simulink model "PubIfDecisionTOS_MDL"  (R2020b)
settings: configuration reference "DspaceConfig" (kept outside this file)
PostLoadFcn:
  | if any(exist('dsrtsu_mdlpostloadfcn', 'file') ~= 0), dsrtsu_mdlpostloadfcn('Execute', bdroot); end
InitFcn:
  | , if any(exist('dsmpb_private', 'file') ~= 0), dsmpb_private('dsmpb_mdlclblib', 'Init', bdroot); end,
undefined symbols (not defined in the file or in its folder): C_TOS_ACCEgoRAxletoFbumplength_m, C_TOS_ACCTargetFront_Flag, C_TOS_AEBJAPedObjDxThre_Val, C_TOS_AEBJAPedObjDyThre_Val, C_TOS_AEBJATargetSize_Val, C_TOS_AEBJAVehObjDxThre_Val, C_TOS_AEBJAVehObjDyThre_Val, C_TOS_AEBJuncPedTargetSize_Val, C_TOS_AEBLatObjDxThre_Val, C_TOS_AEBLatPedDyThre_Val, C_TOS_AEBLatTargetSize_Val, C_TOS_AEBLongTargetInEgoFront_Flag, C_TOS_axAbsGround_Parameter, C_TOS_CameraConfirmedFlag, C_TOS_CNsubjWidth, C_TOS_CurrentLaneCoreMinWidth_Val, C_TOS_CutInProb_Val_Zero, C_TOS_CutOutProb_Val_Zero, C_TOS_D2R_Val, C_TOS_DefaultValueObjectToCenterLine_dy, C_TOS_EgoCarWidth_Val, C_TOS_EgoDxRefPoint_m, C_TOS_EgoRAxletoFbumplength_m, C_TOS_HalfWidthVehicle_Con, C_TOS_HWA_CurrentLaneFlag, C_TOS_HWA_LeftLaneFlag, C_TOS_HWA_MovingDir_Vaild, C_TOS_HWA_MovState_Vaild, C_TOS_HWA_RightLaneFlag, C_TOS_LaneLineCourseErrorFront, C_TOS_LaneLineCourseErrorRear, C_TOS_MotorbikeDefaultWidth_m, C_TOS_NumberOfEffectiveTargets, C_TOS_Obj_Age_Val, C_TOS_Objdx_Constraint_Val, C_TOS_ObjectDefaultWidth_m, C_TOS_ObjInCurrentLane_Val, C_TOS_ObjInCurrentLaneValid, C_TOS_ObjInLeftLaneValid, C_TOS_ObjInRightLaneValid, C_TOS_ObjNotInCurrentLane_Val, C_TOS_ObjNotREElementType, C_TOS_ObjPredictDis_dy_ConstantVal_Zeros, C_TOS_ObjToCenterLine_ConstantVal_Zeros, C_TOS_OFMObjIDInvilad_Val, C_TOS_PIL_LatDisCons_Val_zero, C_TOS_PIL_ObjectCutInFlag_b, C_TOS_PIL_ObjectCutOutFlag_b, C_TOS_PIL_ObjLaneProb_al_Val, C_TOS_PP_ObjFusType_FC_Confirm_b, C_TOS_PP_ObjFusType_FC_FR_Confirm_b, C_TOS_PP_ObjFusType_FR_Confirm_b, C_TOS_RE_80BoolDefault_Val, C_TOS_RE_80Single181Default_Val, C_TOS_RE_80Single255Default_Val, C_TOS_RE_80Uint8Default_Val, C_TOS_RE_D2R, C_TOS_RE_D_180_Val, C_TOS_RE_InvalidObjectID_Val, C_TOS_RE_InvalidTargetChainDir_Val ... (+142)
libraries: simulink x1650, TOS_LIB x361, canfdmsglib x14
(part 35 of 69)

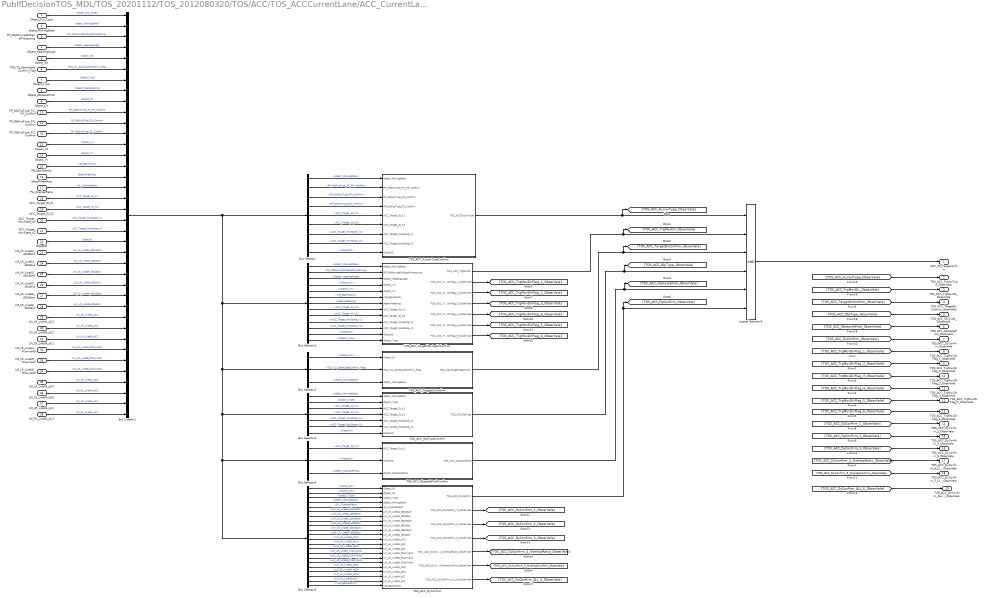
== system PubIfDecisionTOS_MDL/TOS_20201112/TOS_2012080320/TOS/ACC/TOS_ACCCurrentLane/ACC_CurrentLane_Target/TOS_ACC_P0/ACC_P0_Targe/ACC_P0_Targe ==
  Object_Fus_Type : Inport
  object_MovingState : Inport  Port=2
  PP_ObjMovingDirSignalProcessing : Inport  Port=3
  Object_HeadingAngle : Inport  Port=4
  Object_DX : Inport  Port=5
  TOS_TLJ_SameLaneConfirm_Flag : Inport  Port=6
  Object_Type : Inport  Port=7
  Object_ObstacleProb : Inport  Port=8
  Object_DY : Inport  Port=9
  PP_ObjFusType_FC_FR_Confirm : Inport  Port=10
  PP_ObjFusType_FR_Confirm : Inport  Port=11
  PP_ObjFusType_FC_Confirm : Inport  Port=12
  Object_VX : Inport  Port=13
  Object_VY : Inport  Port=14
  VIE_EgoVelocity : Inport  Port=15
  SteerWheelAng : Inport  Port=16
  PIL_OverlapRatio : Inport  Port=17
  ACC_Target_ID_K1 : Inport  Port=18
  ACC_Target_ID_K2 : Inport  Port=19
  ACC_Target_MovState_K1 : Inport  Port=20
  ACC_Target_MovState_K2 : Inport  Port=21
  ObjectID : Inport  Port=22
  LM_LR_Line04_dDisStart : Inport  Port=23
  LM_LR_Line04_dDisEnd : Inport  Port=24
  LM_LR_Line05_dDisStart : Inport  Port=25
  LM_LR_Line05_dDisEnd : Inport  Port=26
  LM_LR_Line06_dDisStart : Inport  Port=27
  LM_LR_Line06_dDisEnd : Inport  Port=28
  LM_LR_Line04_pC2 : Inport  Port=29
  LM_LR_Line05_pC2 : Inport  Port=30
  LM_LR_Line06_pC2 : Inport  Port=31
  LM_LR_Line04_fCamValid : Inport  Port=32
  LM_LR_Line05_fCamValid : Inport  Port=33
  LM_LR_Line06_fCamValid : Inport  Port=34
  LM_LR_Line04_pC0 : Inport  Port=35
  LM_RL_Line04_pC0 : Inport  Port=36
  LM_LR_Line04_pC1 : Inport  Port=37
  LM_RL_Line04_pC1 : Inport  Port=38
  Bus Creator1 : BusCreator  Inputs=38
  Bus Selector : BusSelector  OutputSignals=object_MovingState,PP_ObjFusType_FC_FR_Confirm,PP_ObjFusType_FR_Confirm,PP_ObjFusType_FC_Confirm,ACC_Target_ID_K1,ACC_Target_ID_K2,ACC_Target_MovState_K1,ACC_Target_MovState_K2,ObjectID
  Bus Selector1 : BusSelector  OutputSignals=object_MovingState,PP_ObjMovingDirSignalProcessing,Object_HeadingAngle,Object_VX,Object_VY,VIE_EgoVelocity,SteerWheelAng,ACC_Target_ID_K1,ACC_Target_ID_K2,ACC_Target_MovState_K1,ACC_Target_MovState_K2,ObjectID,Object_Type
  Bus Selector2 : BusSelector  OutputSignals=Object_DX,TOS_TLJ_SameLaneConfirm_Flag,object_MovingState
  Bus Selector3 : BusSelector  OutputSignals=object_MovingState,Object_Type,ACC_Target_ID_K1,ACC_Target_ID_K2,ACC_Target_MovState_K1,ACC_Target_MovState_K2,ObjectID
  Bus Selector4 : BusSelector  OutputSignals=ACC_Target_ID_K1,ObjectID,Object_ObstacleProb
  Bus Selector5 : BusSelector  OutputSignals=Object_DY,Object_DX,Object_Type,object_MovingState,PIL_OverlapRatio,LM_LR_Line04_dDisStart,LM_LR_Line04_dDisEnd,LM_LR_Line05_dDisStart,LM_LR_Line05_dDisEnd,LM_LR_Line06_dDisStart,LM_LR_Line06_dDisEnd,LM_LR_Line04_pC2,LM_LR_Line05_pC2,LM_LR_Line06_pC2,LM_LR_Line04_fCamValid,LM_LR_Line05_fCamValid,LM_LR_Line06_fCamValid,LM_LR_Line04_pC0,LM_RL_Line04_pC0,LM_LR_Line04_pC1,LM_RL_Line04_pC1,VIE_EgoVelocity
  Logical Operator4 : Logic  Inputs=6  AllPortsSameDT=off  OutDataTypeStr=boolean
  TOS_ACC_DyConfirm : Subsystem
  TOS_ACC_FusionTypeConfirm : Subsystem
  TOS_ACC_ObjTypeConfirm : Subsystem
  TOS_ACC_ObstacleProbConfirm : Subsystem
  TOS_ACC_TargetDxConfirm : Subsystem
  TOS_ACC_TargetMovingDirConfirm : Subsystem
  ACC_P0_TargeConfirm : Outport
  TOS_ACC_FusionType_ObserVale : Outport  Port=2
  TOS_ACC_TrgMovDir_ObserVale : Outport  Port=3
  TOS_ACC_TargetDxConfirm_ObserVale : Outport  Port=4
  TOS_ACC_ObjType_ObserVale : Outport  Port=5
  TOS_ACC_ObstacleProb_ObserVale : Outport  Port=6
  TOS_ACC_DyConfirm_ObserVale : Outport  Port=7
  TOS_ACC_TrgMovDirFlag_1_ObserVale : Outport  Port=8
  TOS_ACC_TrgMovDirFlag_2_ObserVale : Outport  Port=9
  TOS_ACC_TrgMovDirFlag_3_ObserVale : Outport  Port=10
  TOS_ACC_TrgMovDirFlag_4_ObserVale : Outport  Port=11
  TOS_ACC_TrgMovDirFlag_5_ObserVale : Outport  Port=12
  TOS_ACC_TrgMovDirFlag_6_ObserVale : Outport  Port=13
  TOS_ACC_DyConfirm_1_ObserVale : Outport  Port=14
  TOS_ACC_DyConfirm_2_ObserVale : Outport  Port=15
  TOS_ACC_DyConfirm_3_ObserVale : Outport  Port=16
  TOS_ACC_DyConfirm_4_OverlapRatio_ObserVale : Outport  Port=17
  TOS_ACC_DyConfirm_5_OverlapConfirm_ObserVale : Outport  Port=18
  TOS_ACC_DyConfirm_ALL_6_ObserVale : Outport  Port=19
  wires:
  Bus Selector2/2 -> TOS_ACC_TargetDxConfirm/2(TOS_TLJ_SameLaneConfirm_Flag)  "<TOS_TLJ_SameLaneConfirm_Flag>"
  TOS_ACC_TargetDxConfirm/1(TOS_ACCTargetInEgoFront) -> [TOS_ACC_TargetDxConfirm_ObserVale], Logical Operator4/3
  TOS_ACC_TargetMovingDirConfirm/1(TOS_ACC_TrgMovDir) -> [TOS_ACC_TrgMovDir_ObserVale], Logical Operator4/2
  Bus Selector2/1 -> TOS_ACC_TargetDxConfirm/1(Object_Dx)  "<Object_DX>"
  TOS_ACC_FusionTypeConfirm/1(TOS_ACCFusionType) -> [TOS_ACC_FusionType_ObserVale], Logical Operator4/1
  TOS_ACC_ObjTypeConfirm/1(TOS_ACCObjType) -> Logical Operator4/4, [TOS_ACC_ObjType_ObserVale]
  Logical Operator4/1 -> ACC_P0_TargeConfirm/1
  [TOS_ACC_FusionType_ObserVale] -> TOS_ACC_FusionType_ObserVale/1
  [TOS_ACC_TrgMovDir_ObserVale] -> TOS_ACC_TrgMovDir_ObserVale/1
  [TOS_ACC_TargetDxConfirm_ObserVale] -> TOS_ACC_TargetDxConfirm_ObserVale/1
  [TOS_ACC_ObjType_ObserVale] -> TOS_ACC_ObjType_ObserVale/1
  [TOS_ACC_ObstacleProb_ObserVale] -> TOS_ACC_ObstacleProb_ObserVale/1
  Bus Selector/1 -> TOS_ACC_FusionTypeConfirm/1(object_MovingState)  "<object_MovingState>"
  Bus Selector1/1 -> TOS_ACC_TargetMovingDirConfirm/1(object_MovingState)  "<object_MovingState>"
  Bus Selector4/3 -> TOS_ACC_ObstacleProbConfirm/3(Object_ObstacleProb)  "<Object_ObstacleProb>"
  TOS_ACC_ObstacleProbConfirm/1(TOS_ACC_ObstacleProb) -> Logical Operator4/5, [TOS_ACC_ObstacleProb_ObserVale]
  TOS_ACC_DyConfirm/1(TOS_ACC_DyConfirm) -> [TOS_ACC_DyConfirm_ObserVale], Logical Operator4/6
  [TOS_ACC_DyConfirm_ObserVale] -> TOS_ACC_DyConfirm_ObserVale/1
  Bus Selector/2 -> TOS_ACC_FusionTypeConfirm/2(PP_ObjFusType_FC_FR_Confirm)  "<PP_ObjFusType_FC_FR_Confirm>"
  Bus Selector/3 -> TOS_ACC_FusionTypeConfirm/3(PP_ObjFusType_FR_Confirm)  "<PP_ObjFusType_FR_Confirm>"
  Bus Selector/4 -> TOS_ACC_FusionTypeConfirm/4(PP_ObjFusType_FC_Confirm)  "<PP_ObjFusType_FC_Confirm>"
  [TOS_ACC_DyConfirm_4_OverlapRatio_ObserVale] -> TOS_ACC_DyConfirm_4_OverlapRatio_ObserVale/1
  Bus Selector/5 -> TOS_ACC_FusionTypeConfirm/5(ACC_Target_ID_K1)  "<ACC_Target_ID_K1>"
  Bus Selector/6 -> TOS_ACC_FusionTypeConfirm/6(ACC_Target_ID_K2)  "<ACC_Target_ID_K2>"
  Bus Selector/9 -> TOS_ACC_FusionTypeConfirm/9(ObjectID)  "<ObjectID>"
  Object_DY/1 -> Bus Creator1/9  "Object_DY"
  PP_ObjFusType_FC_Confirm/1 -> Bus Creator1/12  "PP_ObjFusType_FC_Confirm"
  PP_ObjFusType_FR_Confirm/1 -> Bus Creator1/11  "PP_ObjFusType_FR_Confirm"
  SteerWheelAng/1 -> Bus Creator1/16  "SteerWheelAng"
  PIL_OverlapRatio/1 -> Bus Creator1/17  "PIL_OverlapRatio"
  ACC_Target_MovState_K1/1 -> Bus Creator1/20  "ACC_Target_MovState_K1"
  ACC_Target_ID_K2/1 -> Bus Creator1/19  "ACC_Target_ID_K2"
  Object_DX/1 -> Bus Creator1/5  "Object_DX"
  Object_ObstacleProb/1 -> Bus Creator1/8  "Object_ObstacleProb"
  ObjectID/1 -> Bus Creator1/22  "ObjectID"
  PP_ObjMovingDirSignalProcessing/1 -> Bus Creator1/3  "PP_ObjMovingDirSignalProcessing"
  VIE_EgoVelocity/1 -> Bus Creator1/15  "VIE_EgoVelocity"
  ACC_Target_ID_K1/1 -> Bus Creator1/18  "ACC_Target_ID_K1"
  Object_HeadingAngle/1 -> Bus Creator1/4  "Object_HeadingAngle"
  PP_ObjFusType_FC_FR_Confirm/1 -> Bus Creator1/10  "PP_ObjFusType_FC_FR_Confirm"
  object_MovingState/1 -> Bus Creator1/2  "object_MovingState"
  ACC_Target_MovState_K2/1 -> Bus Creator1/21  "ACC_Target_MovState_K2"
  Object_VY/1 -> Bus Creator1/14  "Object_VY"
  Object_Fus_Type/1 -> Bus Creator1/1  "Object_Fus_Type1"
  Object_Type/1 -> Bus Creator1/7  "Object_Type"
  Object_VX/1 -> Bus Creator1/13  "Object_VX"
  TOS_TLJ_SameLaneConfirm_Flag/1 -> Bus Creator1/6  "TOS_TLJ_SameLaneConfirm_Flag"
  Bus Creator1/1 -> Bus Selector5/1, Bus Selector4/1, Bus Selector3/1, Bus Selector2/1, Bus Selector1/1, Bus Selector/1
  Bus Selector/7 -> TOS_ACC_FusionTypeConfirm/7(ACC_Target_MovState_K1)  "<ACC_Target_MovState_K1>"
  Bus Selector/8 -> TOS_ACC_FusionTypeConfirm/8(ACC_Target_MovState_K2)  "<ACC_Target_MovState_K2>"
  Bus Selector1/2 -> TOS_ACC_TargetMovingDirConfirm/2(PP_ObjMovingDirSignalProcessing)  "<PP_ObjMovingDirSignalProcessing>"
  Bus Selector1/3 -> TOS_ACC_TargetMovingDirConfirm/3(Object_HeadingAngle)  "<Object_HeadingAngle>"
  Bus Selector1/4 -> TOS_ACC_TargetMovingDirConfirm/4(Object_VX)  "<Object_VX>"
  Bus Selector1/5 -> TOS_ACC_TargetMovingDirConfirm/5(Object_VY)  "<Object_VY>"
  Bus Selector1/6 -> TOS_ACC_TargetMovingDirConfirm/6(VIE_EgoVelocity)  "<VIE_EgoVelocity>"
  Bus Selector1/7 -> TOS_ACC_TargetMovingDirConfirm/7(SteerWheelAng)  "<SteerWheelAng>"
  Bus Selector3/1 -> TOS_ACC_ObjTypeConfirm/1(object_MovingState)  "<object_MovingState>"
  Bus Selector3/2 -> TOS_ACC_ObjTypeConfirm/2(Object_Type)  "<Object_Type>"
  Bus Selector5/1 -> TOS_ACC_DyConfirm/1(Object_DY)  "<Object_DY>"
  Bus Selector5/2 -> TOS_ACC_DyConfirm/2(Object_DX)  "<Object_DX>"
  Bus Selector5/3 -> TOS_ACC_DyConfirm/3(Object_Type)  "<Object_Type>"
  Bus Selector4/1 -> TOS_ACC_ObstacleProbConfirm/1(ACC_Target_ID_K1)  "<ACC_Target_ID_K1>"
  Bus Selector4/2 -> TOS_ACC_ObstacleProbConfirm/2(ObjectID)  "<ObjectID>"
  Bus Selector3/3 -> TOS_ACC_ObjTypeConfirm/3(ACC_Target_ID_K1)  "<ACC_Target_ID_K1>"
  Bus Selector3/4 -> TOS_ACC_ObjTypeConfirm/4(ACC_Target_ID_K2)  "<ACC_Target_ID_K2>"
  Bus Selector3/5 -> TOS_ACC_ObjTypeConfirm/5(ACC_Target_MovState_K1)  "<ACC_Target_MovState_K1>"
  Bus Selector3/6 -> TOS_ACC_ObjTypeConfirm/6(ACC_Target_MovState_K2)  "<ACC_Target_MovState_K2>"
  Bus Selector3/7 -> TOS_ACC_ObjTypeConfirm/7(ObjectID)  "<ObjectID>"
  Bus Selector1/8 -> TOS_ACC_TargetMovingDirConfirm/8(ACC_Target_ID_K1)  "<ACC_Target_ID_K1>"
  Bus Selector1/9 -> TOS_ACC_TargetMovingDirConfirm/9(ACC_Target_ID_K2)  "<ACC_Target_ID_K2>"
  Bus Selector1/10 -> TOS_ACC_TargetMovingDirConfirm/10(ACC_Target_MovState_K1)  "<ACC_Target_MovState_K1>"
  Bus Selector1/11 -> TOS_ACC_TargetMovingDirConfirm/11(ACC_Target_MovState_K2)  "<ACC_Target_MovState_K2>"
  Bus Selector1/12 -> TOS_ACC_TargetMovingDirConfirm/12(ObjectID)  "<ObjectID>"
  [TOS_ACC_TrgMovDirFlag_1_ObserVale] -> TOS_ACC_TrgMovDirFlag_1_ObserVale/1
  [TOS_ACC_TrgMovDirFlag_3_ObserVale] -> TOS_ACC_TrgMovDirFlag_3_ObserVale/1
  [TOS_ACC_TrgMovDirFlag_2_ObserVale] -> TOS_ACC_TrgMovDirFlag_2_ObserVale/1
  [TOS_ACC_TrgMovDirFlag_5_ObserVale] -> TOS_ACC_TrgMovDirFlag_5_ObserVale/1
  [TOS_ACC_TrgMovDirFlag_4_ObserVale] -> TOS_ACC_TrgMovDirFlag_4_ObserVale/1
  TOS_ACC_TargetMovingDirConfirm/2(TOS_ACC_TrgMovDirFlag_1_ObserVale) -> [TOS_ACC_TrgMovDirFlag_1_ObserVale]
  TOS_ACC_TargetMovingDirConfirm/3(TOS_ACC_TrgMovDirFlag_2_ObserVale) -> [TOS_ACC_TrgMovDirFlag_2_ObserVale]
  TOS_ACC_TargetMovingDirConfirm/4(TOS_ACC_TrgMovDirFlag_3_ObserVale) -> [TOS_ACC_TrgMovDirFlag_3_ObserVale]
  TOS_ACC_TargetMovingDirConfirm/5(TOS_ACC_TrgMovDirFlag_4_ObserVale) -> [TOS_ACC_TrgMovDirFlag_4_ObserVale]
  TOS_ACC_TargetMovingDirConfirm/6(TOS_ACC_TrgMovDirFlag_5_ObserVale) -> [TOS_ACC_TrgMovDirFlag_5_ObserVale]
  Bus Selector2/3 -> TOS_ACC_TargetDxConfirm/3(object_MovingState)  "<object_MovingState>"
  Bus Selector5/4 -> TOS_ACC_DyConfirm/4(object_MovingState)  "<object_MovingState>"
  [TOS_ACC_DyConfirm_2_ObserVale] -> TOS_ACC_DyConfirm_2_ObserVale/1
  [TOS_ACC_DyConfirm_3_ObserVale] -> TOS_ACC_DyConfirm_3_ObserVale/1
  [TOS_ACC_DyConfirm_1_ObserVale] -> TOS_ACC_DyConfirm_1_ObserVale/1
  TOS_ACC_DyConfirm/2(TOS_ACC_DyConfirm_1_ObserVale) -> [TOS_ACC_DyConfirm_1_ObserVale]
  TOS_ACC_DyConfirm/3(TOS_ACC_DyConfirm_2_ObserVale) -> [TOS_ACC_DyConfirm_2_ObserVale]
  TOS_ACC_DyConfirm/4(TOS_ACC_DyConfirm_3_ObserVale) -> [TOS_ACC_DyConfirm_3_ObserVale]
  TOS_ACC_TargetMovingDirConfirm/7(TOS_ACC_TrgMovDirFlag_6_ObserVale) -> [TOS_ACC_TrgMovDirFlag_6_ObserVale]
  [TOS_ACC_TrgMovDirFlag_6_ObserVale] -> TOS_ACC_TrgMovDirFlag_6_ObserVale/1
  Bus Selector5/5 -> TOS_ACC_DyConfirm/5(PIL_OverlapRatio)  "<PIL_OverlapRatio>"
  TOS_ACC_DyConfirm/5(TOS_ACC_DyConfirm_4_OverlapRatio_ObserVale) -> [TOS_ACC_DyConfirm_4_OverlapRatio_ObserVale]
  Bus Selector1/13 -> TOS_ACC_TargetMovingDirConfirm/13(Object_Type)  "<Object_Type>"
  LM_LR_Line04_dDisStart/1 -> Bus Creator1/23  "LM_LR_Line04_dDisStart"
  LM_LR_Line04_dDisEnd/1 -> Bus Creator1/24  "LM_LR_Line04_dDisEnd"
  LM_LR_Line05_dDisStart/1 -> Bus Creator1/25  "LM_LR_Line05_dDisStart"
  LM_LR_Line05_dDisEnd/1 -> Bus Creator1/26  "LM_LR_Line05_dDisEnd"
  LM_LR_Line06_dDisStart/1 -> Bus Creator1/27  "LM_LR_Line06_dDisStart"
  LM_LR_Line06_dDisEnd/1 -> Bus Creator1/28  "LM_LR_Line06_dDisEnd"
  LM_LR_Line04_pC2/1 -> Bus Creator1/29  "LM_LR_Line04_pC2"
  LM_LR_Line05_pC2/1 -> Bus Creator1/30  "LM_LR_Line05_pC2"
  LM_LR_Line06_pC2/1 -> Bus Creator1/31  "LM_LR_Line06_pC2"
  Bus Selector5/6 -> TOS_ACC_DyConfirm/6(LM_LR_Line04_dDisStart)  "<LM_LR_Line04_dDisStart>"
  Bus Selector5/7 -> TOS_ACC_DyConfirm/7(LM_LR_Line04_dDisEnd)  "<LM_LR_Line04_dDisEnd>"
  Bus Selector5/8 -> TOS_ACC_DyConfirm/8(LM_LR_Line05_dDisStart)  "<LM_LR_Line05_dDisStart>"
  Bus Selector5/9 -> TOS_ACC_DyConfirm/9(LM_LR_Line05_dDisEnd)  "<LM_LR_Line05_dDisEnd>"
  Bus Selector5/10 -> TOS_ACC_DyConfirm/10(LM_LR_Line06_dDisStart)  "<LM_LR_Line06_dDisStart>"
  Bus Selector5/11 -> TOS_ACC_DyConfirm/11(LM_LR_Line06_dDisEnd)  "<LM_LR_Line06_dDisEnd>"
  Bus Selector5/12 -> TOS_ACC_DyConfirm/12(LM_LR_Line04_pC2)  "<LM_LR_Line04_pC2>"
  Bus Selector5/13 -> TOS_ACC_DyConfirm/13(LM_LR_Line05_pC2)  "<LM_LR_Line05_pC2>"
  Bus Selector5/14 -> TOS_ACC_DyConfirm/14(LM_LR_Line06_pC2)  "<LM_LR_Line06_pC2>"
  LM_LR_Line04_fCamValid/1 -> Bus Creator1/32  "LM_LR_Line04_fCamValid"
  LM_LR_Line05_fCamValid/1 -> Bus Creator1/33  "LM_LR_Line05_fCamValid"
  LM_LR_Line06_fCamValid/1 -> Bus Creator1/34  "LM_LR_Line06_fCamValid"
  Bus Selector5/15 -> TOS_ACC_DyConfirm/15(LM_LR_Line04_fCamValid)  "<LM_LR_Line04_fCamValid>"
  Bus Selector5/16 -> TOS_ACC_DyConfirm/16(LM_LR_Line05_fCamValid)  "<LM_LR_Line05_fCamValid>"
  Bus Selector5/17 -> TOS_ACC_DyConfirm/17(LM_LR_Line06_fCamValid)  "<LM_LR_Line06_fCamValid>"
  [TOS_ACC_DyConfirm_5_OverlapConfirm_ObserVale] -> TOS_ACC_DyConfirm_5_OverlapConfirm_ObserVale/1
  TOS_ACC_DyConfirm/6(TOS_ACC_DyConfirm_5_OverlapConfirm_ObserVale) -> [TOS_ACC_DyConfirm_5_OverlapConfirm_ObserVale]
  TOS_ACC_DyConfirm/7(TOS_ACC_DyConfirm_ALL_6_ObserVale) -> [TOS_ACC_DyConfirm_ALL_6_ObserVale]
  [TOS_ACC_DyConfirm_ALL_6_ObserVale] -> TOS_ACC_DyConfirm_ALL_6_ObserVale/1
  LM_LR_Line04_pC0/1 -> Bus Creator1/35  "LM_LR_Line04_pC0"
  LM_RL_Line04_pC0/1 -> Bus Creator1/36  "LM_RL_Line04_pC0"
  Bus Selector5/18 -> TOS_ACC_DyConfirm/18(LM_LR_Line04_pC0)  "<LM_LR_Line04_pC0>"
  Bus Selector5/19 -> TOS_ACC_DyConfirm/19(LM_RL_Line04_pC0)  "<LM_RL_Line04_pC0>"
  LM_LR_Line04_pC1/1 -> Bus Creator1/37  "LM_LR_Line04_pC1"
  LM_RL_Line04_pC1/1 -> Bus Creator1/38  "LM_RL_Line04_pC1"
  Bus Selector5/20 -> TOS_ACC_DyConfirm/20(LM_LR_Line04_pC1)  "<LM_LR_Line04_pC1>"
  Bus Selector5/21 -> TOS_ACC_DyConfirm/21(LM_RL_Line04_pC1)  "<LM_RL_Line04_pC1>"
  Bus Selector5/22 -> TOS_ACC_DyConfirm/22(VIE_EgoVelocity)  "<VIE_EgoVelocity>"

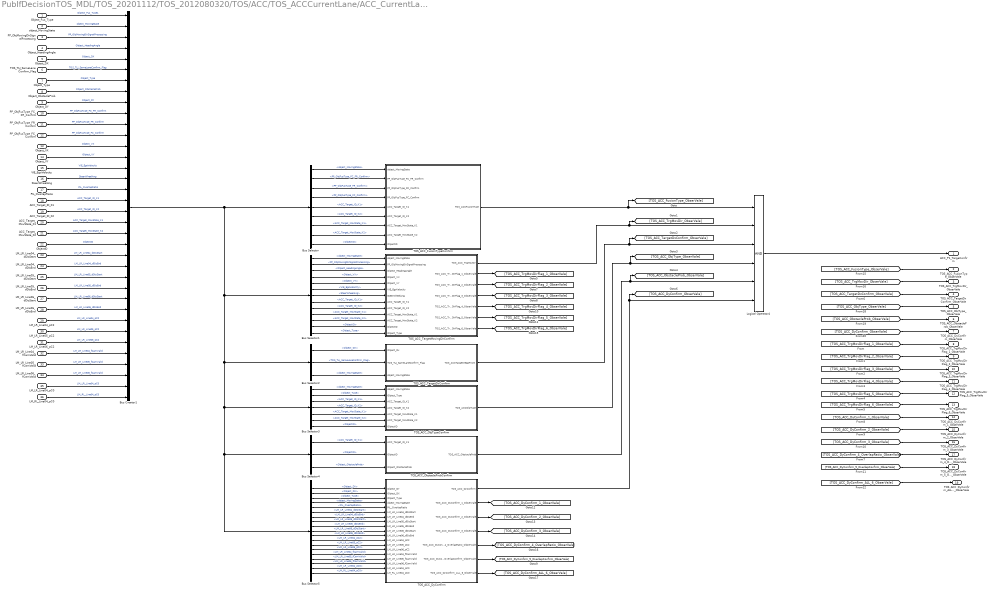
== system PubIfDecisionTOS_MDL/TOS_20201112/TOS_2012080320/TOS/ACC/TOS_ACCCurrentLane/ACC_CurrentLane_Target/TOS_ACC_P1/ACC_P1_Targe/ACC_P1_Targe ==
  Object_Fus_Type : Inport
  object_MovingState : Inport  Port=2
  PP_ObjMovingDirSignalProcessing : Inport  Port=3
  Object_HeadingAngle : Inport  Port=4
  Object_DX : Inport  Port=5
  TOS_TLJ_SameLaneConfirm_Flag : Inport  Port=6
  Object_Type : Inport  Port=7
  Object_ObstacleProb : Inport  Port=8
  Object_DY : Inport  Port=9
  PP_ObjFusType_FC_FR_Confirm : Inport  Port=10
  PP_ObjFusType_FR_Confirm : Inport  Port=11
  PP_ObjFusType_FC_Confirm : Inport  Port=12
  Object_VX : Inport  Port=13
  Object_VY : Inport  Port=14
  VIE_EgoVelocity : Inport  Port=15
  SteerWheelAng : Inport  Port=16
  PIL_OverlapRatio : Inport  Port=17
  ACC_Target_ID_K1 : Inport  Port=18
  ACC_Target_ID_K2 : Inport  Port=19
  ACC_Target_MovState_K1 : Inport  Port=20
  ACC_Target_MovState_K2 : Inport  Port=21
  ObjectID : Inport  Port=22
  LM_LR_Line04_dDisStart : Inport  Port=23
  LM_LR_Line04_dDisEnd : Inport  Port=24
  LM_LR_Line05_dDisStart : Inport  Port=25
  LM_LR_Line05_dDisEnd : Inport  Port=26
  LM_LR_Line06_dDisStart : Inport  Port=27
  LM_LR_Line06_dDisEnd : Inport  Port=28
  LM_LR_Line04_pC2 : Inport  Port=29
  LM_LR_Line05_pC2 : Inport  Port=30
  LM_LR_Line06_pC2 : Inport  Port=31
  LM_LR_Line04_fCamValid : Inport  Port=32
  LM_LR_Line05_fCamValid : Inport  Port=33
  LM_LR_Line06_fCamValid : Inport  Port=34
  LM_LR_Line04_pC0 : Inport  Port=35
  LM_RL_Line04_pC0 : Inport  Port=36
  Bus Creator1 : BusCreator  Inputs=36
  Bus Selector : BusSelector  OutputSignals=object_MovingState,PP_ObjFusType_FC_FR_Confirm,PP_ObjFusType_FR_Confirm,PP_ObjFusType_FC_Confirm,ACC_Target_ID_K1,ACC_Target_ID_K2,ACC_Target_MovState_K1,ACC_Target_MovState_K2,ObjectID
  Bus Selector1 : BusSelector  OutputSignals=object_MovingState,PP_ObjMovingDirSignalProcessing,Object_HeadingAngle,Object_VX,Object_VY,VIE_EgoVelocity,SteerWheelAng,ACC_Target_ID_K1,ACC_Target_ID_K2,ACC_Target_MovState_K1,ACC_Target_MovState_K2,ObjectID,Object_Type
  Bus Selector2 : BusSelector  OutputSignals=Object_DX,TOS_TLJ_SameLaneConfirm_Flag,object_MovingState
  Bus Selector3 : BusSelector  OutputSignals=object_MovingState,Object_Type,ACC_Target_ID_K1,ACC_Target_ID_K2,ACC_Target_MovState_K1,ACC_Target_MovState_K2,ObjectID
  Bus Selector4 : BusSelector  OutputSignals=ACC_Target_ID_K1,ObjectID,Object_ObstacleProb
  Bus Selector5 : BusSelector  OutputSignals=Object_DY,Object_DX,Object_Type,object_MovingState,PIL_OverlapRatio,LM_LR_Line04_dDisStart,LM_LR_Line04_dDisEnd,LM_LR_Line05_dDisStart,LM_LR_Line05_dDisEnd,LM_LR_Line06_dDisStart,LM_LR_Line06_dDisEnd,LM_LR_Line04_pC2,LM_LR_Line05_pC2,LM_LR_Line06_pC2,LM_LR_Line04_fCamValid,LM_LR_Line05_fCamValid,LM_LR_Line06_fCamValid,LM_LR_Line04_pC0,LM_RL_Line04_pC0
  Logical Operator4 : Logic  Inputs=6  AllPortsSameDT=off  OutDataTypeStr=boolean
  TOS_ACC_DyConfirm : Subsystem
  TOS_ACC_FusionTypeConfirm : Subsystem
  TOS_ACC_ObjTypeConfirm : Subsystem
  TOS_ACC_ObstacleProbConfirm : Subsystem
  TOS_ACC_TargetDxConfirm : Subsystem
  TOS_ACC_TargetMovingDirConfirm : Subsystem
  ACC_P1_TargeConfirm : Outport
  TOS_ACC_FusionType_ObserVale : Outport  Port=2
  TOS_ACC_TrgMovDir_ObserVale : Outport  Port=3
  TOS_ACC_TargetDxConfirm_ObserVale : Outport  Port=4
  TOS_ACC_ObjType_ObserVale : Outport  Port=5
  TOS_ACC_ObstacleProb_ObserVale : Outport  Port=6
  TOS_ACC_DyConfirm_ObserVale : Outport  Port=7
  TOS_ACC_TrgMovDirFlag_1_ObserVale : Outport  Port=8
  TOS_ACC_TrgMovDirFlag_2_ObserVale : Outport  Port=9
  TOS_ACC_TrgMovDirFlag_3_ObserVale : Outport  Port=10
  TOS_ACC_TrgMovDirFlag_4_ObserVale : Outport  Port=11
  TOS_ACC_TrgMovDirFlag_5_ObserVale : Outport  Port=12
  TOS_ACC_TrgMovDirFlag_6_ObserVale : Outport  Port=13
  TOS_ACC_DyConfirm_1_ObserVale : Outport  Port=14
  TOS_ACC_DyConfirm_2_ObserVale : Outport  Port=15
  TOS_ACC_DyConfirm_3_ObserVale : Outport  Port=16
  TOS_ACC_DyConfirm_4_OverlapRatio_ObserVale : Outport  Port=17
  TOS_ACC_DyConfirm_5_OverlapConfirm_ObserVale : Outport  Port=18
  TOS_ACC_DyConfirm_ALL_6_ObserVale : Outport  Port=19
  wires:
  Bus Selector5/19 -> TOS_ACC_DyConfirm/19(LM_RL_Line04_pC0)  "<LM_RL_Line04_pC0>"
  Bus Selector5/18 -> TOS_ACC_DyConfirm/18(LM_LR_Line04_pC0)  "<LM_LR_Line04_pC0>"
  LM_RL_Line04_pC0/1 -> Bus Creator1/36  "LM_RL_Line04_pC0"
  LM_LR_Line04_pC0/1 -> Bus Creator1/35  "LM_LR_Line04_pC0"
  [TOS_ACC_DyConfirm_ALL_6_ObserVale] -> TOS_ACC_DyConfirm_ALL_6_ObserVale/1
  TOS_ACC_DyConfirm/7(TOS_ACC_DyConfirm_ALL_6_ObserVale) -> [TOS_ACC_DyConfirm_ALL_6_ObserVale]
  TOS_ACC_DyConfirm/6(TOS_ACC_DyConfirm_5_OverlapConfirm_ObserVale) -> [TOS_ACC_DyConfirm_5_OverlapConfirm_ObserVale]
  [TOS_ACC_DyConfirm_5_OverlapConfirm_ObserVale] -> TOS_ACC_DyConfirm_5_OverlapConfirm_ObserVale/1
  Bus Selector5/17 -> TOS_ACC_DyConfirm/17(LM_LR_Line06_fCamValid)  "<LM_LR_Line06_fCamValid>"
  Bus Selector5/16 -> TOS_ACC_DyConfirm/16(LM_LR_Line05_fCamValid)  "<LM_LR_Line05_fCamValid>"
  Bus Selector5/15 -> TOS_ACC_DyConfirm/15(LM_LR_Line04_fCamValid)  "<LM_LR_Line04_fCamValid>"
  LM_LR_Line06_fCamValid/1 -> Bus Creator1/34  "LM_LR_Line06_fCamValid"
  LM_LR_Line05_fCamValid/1 -> Bus Creator1/33  "LM_LR_Line05_fCamValid"
  LM_LR_Line04_fCamValid/1 -> Bus Creator1/32  "LM_LR_Line04_fCamValid"
  Bus Selector5/14 -> TOS_ACC_DyConfirm/14(LM_LR_Line06_pC2)  "<LM_LR_Line06_pC2>"
  Bus Selector5/13 -> TOS_ACC_DyConfirm/13(LM_LR_Line05_pC2)  "<LM_LR_Line05_pC2>"
  Bus Selector5/12 -> TOS_ACC_DyConfirm/12(LM_LR_Line04_pC2)  "<LM_LR_Line04_pC2>"
  Bus Selector5/11 -> TOS_ACC_DyConfirm/11(LM_LR_Line06_dDisEnd)  "<LM_LR_Line06_dDisEnd>"
  Bus Selector5/10 -> TOS_ACC_DyConfirm/10(LM_LR_Line06_dDisStart)  "<LM_LR_Line06_dDisStart>"
  Bus Selector5/9 -> TOS_ACC_DyConfirm/9(LM_LR_Line05_dDisEnd)  "<LM_LR_Line05_dDisEnd>"
  Bus Selector5/8 -> TOS_ACC_DyConfirm/8(LM_LR_Line05_dDisStart)  "<LM_LR_Line05_dDisStart>"
  Bus Selector5/7 -> TOS_ACC_DyConfirm/7(LM_LR_Line04_dDisEnd)  "<LM_LR_Line04_dDisEnd>"
  Bus Selector5/6 -> TOS_ACC_DyConfirm/6(LM_LR_Line04_dDisStart)  "<LM_LR_Line04_dDisStart>"
  LM_LR_Line06_pC2/1 -> Bus Creator1/31  "LM_LR_Line06_pC2"
  LM_LR_Line05_pC2/1 -> Bus Creator1/30  "LM_LR_Line05_pC2"
  LM_LR_Line04_pC2/1 -> Bus Creator1/29  "LM_LR_Line04_pC2"
  LM_LR_Line06_dDisEnd/1 -> Bus Creator1/28  "LM_LR_Line06_dDisEnd"
  LM_LR_Line06_dDisStart/1 -> Bus Creator1/27  "LM_LR_Line06_dDisStart"
  LM_LR_Line05_dDisEnd/1 -> Bus Creator1/26  "LM_LR_Line05_dDisEnd"
  LM_LR_Line05_dDisStart/1 -> Bus Creator1/25  "LM_LR_Line05_dDisStart"
  LM_LR_Line04_dDisEnd/1 -> Bus Creator1/24  "LM_LR_Line04_dDisEnd"
  LM_LR_Line04_dDisStart/1 -> Bus Creator1/23  "LM_LR_Line04_dDisStart"
  Bus Selector1/13 -> TOS_ACC_TargetMovingDirConfirm/13(Object_Type)  "<Object_Type>"
  TOS_ACC_DyConfirm/5(TOS_ACC_DyConfirm_4_OverlapRatio_ObserVale) -> [TOS_ACC_DyConfirm_4_OverlapRatio_ObserVale]
  Bus Selector5/5 -> TOS_ACC_DyConfirm/5(PIL_OverlapRatio)  "<PIL_OverlapRatio>"
  [TOS_ACC_TrgMovDirFlag_6_ObserVale] -> TOS_ACC_TrgMovDirFlag_6_ObserVale/1
  TOS_ACC_TargetMovingDirConfirm/7(TOS_ACC_TrgMovDirFlag_6_ObserVale) -> [TOS_ACC_TrgMovDirFlag_6_ObserVale]
  TOS_ACC_DyConfirm/4(TOS_ACC_DyConfirm_3_ObserVale) -> [TOS_ACC_DyConfirm_3_ObserVale]
  TOS_ACC_DyConfirm/3(TOS_ACC_DyConfirm_2_ObserVale) -> [TOS_ACC_DyConfirm_2_ObserVale]
  TOS_ACC_DyConfirm/2(TOS_ACC_DyConfirm_1_ObserVale) -> [TOS_ACC_DyConfirm_1_ObserVale]
  [TOS_ACC_DyConfirm_1_ObserVale] -> TOS_ACC_DyConfirm_1_ObserVale/1
  [TOS_ACC_DyConfirm_3_ObserVale] -> TOS_ACC_DyConfirm_3_ObserVale/1
  [TOS_ACC_DyConfirm_2_ObserVale] -> TOS_ACC_DyConfirm_2_ObserVale/1
  Bus Selector5/4 -> TOS_ACC_DyConfirm/4(object_MovingState)  "<object_MovingState>"
  Bus Selector2/3 -> TOS_ACC_TargetDxConfirm/3(object_MovingState)  "<object_MovingState>"
  TOS_ACC_TargetMovingDirConfirm/6(TOS_ACC_TrgMovDirFlag_5_ObserVale) -> [TOS_ACC_TrgMovDirFlag_5_ObserVale]
  TOS_ACC_TargetMovingDirConfirm/5(TOS_ACC_TrgMovDirFlag_4_ObserVale) -> [TOS_ACC_TrgMovDirFlag_4_ObserVale]
  TOS_ACC_TargetMovingDirConfirm/4(TOS_ACC_TrgMovDirFlag_3_ObserVale) -> [TOS_ACC_TrgMovDirFlag_3_ObserVale]
  TOS_ACC_TargetMovingDirConfirm/3(TOS_ACC_TrgMovDirFlag_2_ObserVale) -> [TOS_ACC_TrgMovDirFlag_2_ObserVale]
  TOS_ACC_TargetMovingDirConfirm/2(TOS_ACC_TrgMovDirFlag_1_ObserVale) -> [TOS_ACC_TrgMovDirFlag_1_ObserVale]
  [TOS_ACC_TrgMovDirFlag_4_ObserVale] -> TOS_ACC_TrgMovDirFlag_4_ObserVale/1
  [TOS_ACC_TrgMovDirFlag_5_ObserVale] -> TOS_ACC_TrgMovDirFlag_5_ObserVale/1
  [TOS_ACC_TrgMovDirFlag_2_ObserVale] -> TOS_ACC_TrgMovDirFlag_2_ObserVale/1
  [TOS_ACC_TrgMovDirFlag_3_ObserVale] -> TOS_ACC_TrgMovDirFlag_3_ObserVale/1
  [TOS_ACC_TrgMovDirFlag_1_ObserVale] -> TOS_ACC_TrgMovDirFlag_1_ObserVale/1
  Bus Selector1/12 -> TOS_ACC_TargetMovingDirConfirm/12(ObjectID)  "<ObjectID>"
  Bus Selector1/11 -> TOS_ACC_TargetMovingDirConfirm/11(ACC_Target_MovState_K2)  "<ACC_Target_MovState_K2>"
  Bus Selector1/10 -> TOS_ACC_TargetMovingDirConfirm/10(ACC_Target_MovState_K1)  "<ACC_Target_MovState_K1>"
  Bus Selector1/9 -> TOS_ACC_TargetMovingDirConfirm/9(ACC_Target_ID_K2)  "<ACC_Target_ID_K2>"
  Bus Selector1/8 -> TOS_ACC_TargetMovingDirConfirm/8(ACC_Target_ID_K1)  "<ACC_Target_ID_K1>"
  Bus Selector3/7 -> TOS_ACC_ObjTypeConfirm/7(ObjectID)  "<ObjectID>"
  Bus Selector3/6 -> TOS_ACC_ObjTypeConfirm/6(ACC_Target_MovState_K2)  "<ACC_Target_MovState_K2>"
  Bus Selector3/5 -> TOS_ACC_ObjTypeConfirm/5(ACC_Target_MovState_K1)  "<ACC_Target_MovState_K1>"
  Bus Selector3/4 -> TOS_ACC_ObjTypeConfirm/4(ACC_Target_ID_K2)  "<ACC_Target_ID_K2>"
  Bus Selector3/3 -> TOS_ACC_ObjTypeConfirm/3(ACC_Target_ID_K1)  "<ACC_Target_ID_K1>"
  Bus Selector4/2 -> TOS_ACC_ObstacleProbConfirm/2(ObjectID)  "<ObjectID>"
  Bus Selector4/1 -> TOS_ACC_ObstacleProbConfirm/1(ACC_Target_ID_K1)  "<ACC_Target_ID_K1>"
  Bus Selector5/3 -> TOS_ACC_DyConfirm/3(Object_Type)  "<Object_Type>"
  Bus Selector5/2 -> TOS_ACC_DyConfirm/2(Object_DX)  "<Object_DX>"
  Bus Selector5/1 -> TOS_ACC_DyConfirm/1(Object_DY)  "<Object_DY>"
  Bus Selector3/2 -> TOS_ACC_ObjTypeConfirm/2(Object_Type)  "<Object_Type>"
  Bus Selector3/1 -> TOS_ACC_ObjTypeConfirm/1(object_MovingState)  "<object_MovingState>"
  Bus Selector1/7 -> TOS_ACC_TargetMovingDirConfirm/7(SteerWheelAng)  "<SteerWheelAng>"
  Bus Selector1/6 -> TOS_ACC_TargetMovingDirConfirm/6(VIE_EgoVelocity)  "<VIE_EgoVelocity>"
  Bus Selector1/5 -> TOS_ACC_TargetMovingDirConfirm/5(Object_VY)  "<Object_VY>"
  Bus Selector1/4 -> TOS_ACC_TargetMovingDirConfirm/4(Object_VX)  "<Object_VX>"
  Bus Selector1/3 -> TOS_ACC_TargetMovingDirConfirm/3(Object_HeadingAngle)  "<Object_HeadingAngle>"
  Bus Selector1/2 -> TOS_ACC_TargetMovingDirConfirm/2(PP_ObjMovingDirSignalProcessing)  "<PP_ObjMovingDirSignalProcessing>"
  Bus Selector/8 -> TOS_ACC_FusionTypeConfirm/8(ACC_Target_MovState_K2)  "<ACC_Target_MovState_K2>"
  Bus Selector/7 -> TOS_ACC_FusionTypeConfirm/7(ACC_Target_MovState_K1)  "<ACC_Target_MovState_K1>"
  Bus Creator1/1 -> Bus Selector/1, Bus Selector1/1, Bus Selector2/1, Bus Selector3/1, Bus Selector4/1, Bus Selector5/1
  TOS_TLJ_SameLaneConfirm_Flag/1 -> Bus Creator1/6  "TOS_TLJ_SameLaneConfirm_Flag"
  Object_VX/1 -> Bus Creator1/13  "Object_VX"
  Object_Type/1 -> Bus Creator1/7  "Object_Type"
  Object_Fus_Type/1 -> Bus Creator1/1  "Object_Fus_Type1"
  Object_VY/1 -> Bus Creator1/14  "Object_VY"
  ACC_Target_MovState_K2/1 -> Bus Creator1/21  "ACC_Target_MovState_K2"
  object_MovingState/1 -> Bus Creator1/2  "object_MovingState"
  PP_ObjFusType_FC_FR_Confirm/1 -> Bus Creator1/10  "PP_ObjFusType_FC_FR_Confirm"
  Object_HeadingAngle/1 -> Bus Creator1/4  "Object_HeadingAngle"
  ACC_Target_ID_K1/1 -> Bus Creator1/18  "ACC_Target_ID_K1"
  VIE_EgoVelocity/1 -> Bus Creator1/15  "VIE_EgoVelocity"
  PP_ObjMovingDirSignalProcessing/1 -> Bus Creator1/3  "PP_ObjMovingDirSignalProcessing"
  ObjectID/1 -> Bus Creator1/22  "ObjectID"
  Object_ObstacleProb/1 -> Bus Creator1/8  "Object_ObstacleProb"
  Object_DX/1 -> Bus Creator1/5  "Object_DX"
  ACC_Target_ID_K2/1 -> Bus Creator1/19  "ACC_Target_ID_K2"
  ACC_Target_MovState_K1/1 -> Bus Creator1/20  "ACC_Target_MovState_K1"
  PIL_OverlapRatio/1 -> Bus Creator1/17  "PIL_OverlapRatio"
  SteerWheelAng/1 -> Bus Creator1/16  "SteerWheelAng"
  PP_ObjFusType_FR_Confirm/1 -> Bus Creator1/11  "PP_ObjFusType_FR_Confirm"
  PP_ObjFusType_FC_Confirm/1 -> Bus Creator1/12  "PP_ObjFusType_FC_Confirm"
  Object_DY/1 -> Bus Creator1/9  "Object_DY"
  Bus Selector/9 -> TOS_ACC_FusionTypeConfirm/9(ObjectID)  "<ObjectID>"
  Bus Selector/6 -> TOS_ACC_FusionTypeConfirm/6(ACC_Target_ID_K2)  "<ACC_Target_ID_K2>"
  Bus Selector/5 -> TOS_ACC_FusionTypeConfirm/5(ACC_Target_ID_K1)  "<ACC_Target_ID_K1>"
  [TOS_ACC_DyConfirm_4_OverlapRatio_ObserVale] -> TOS_ACC_DyConfirm_4_OverlapRatio_ObserVale/1
  Bus Selector/4 -> TOS_ACC_FusionTypeConfirm/4(PP_ObjFusType_FC_Confirm)  "<PP_ObjFusType_FC_Confirm>"
  Bus Selector/3 -> TOS_ACC_FusionTypeConfirm/3(PP_ObjFusType_FR_Confirm)  "<PP_ObjFusType_FR_Confirm>"
  Bus Selector/2 -> TOS_ACC_FusionTypeConfirm/2(PP_ObjFusType_FC_FR_Confirm)  "<PP_ObjFusType_FC_FR_Confirm>"
  [TOS_ACC_DyConfirm_ObserVale] -> TOS_ACC_DyConfirm_ObserVale/1
  TOS_ACC_DyConfirm/1(TOS_ACC_DyConfirm) -> Logical Operator4/6, [TOS_ACC_DyConfirm_ObserVale]
  TOS_ACC_ObstacleProbConfirm/1(TOS_ACC_ObstacleProb) -> [TOS_ACC_ObstacleProb_ObserVale], Logical Operator4/5
  Bus Selector4/3 -> TOS_ACC_ObstacleProbConfirm/3(Object_ObstacleProb)  "<Object_ObstacleProb>"
  Bus Selector1/1 -> TOS_ACC_TargetMovingDirConfirm/1(object_MovingState)  "<object_MovingState>"
  Bus Selector/1 -> TOS_ACC_FusionTypeConfirm/1(object_MovingState)  "<object_MovingState>"
  [TOS_ACC_ObstacleProb_ObserVale] -> TOS_ACC_ObstacleProb_ObserVale/1
  [TOS_ACC_ObjType_ObserVale] -> TOS_ACC_ObjType_ObserVale/1
  [TOS_ACC_TargetDxConfirm_ObserVale] -> TOS_ACC_TargetDxConfirm_ObserVale/1
  [TOS_ACC_TrgMovDir_ObserVale] -> TOS_ACC_TrgMovDir_ObserVale/1
  [TOS_ACC_FusionType_ObserVale] -> TOS_ACC_FusionType_ObserVale/1
  Logical Operator4/1 -> ACC_P1_TargeConfirm/1
  TOS_ACC_ObjTypeConfirm/1(TOS_ACCObjType) -> [TOS_ACC_ObjType_ObserVale], Logical Operator4/4
  TOS_ACC_FusionTypeConfirm/1(TOS_ACCFusionType) -> Logical Operator4/1, [TOS_ACC_FusionType_ObserVale]
  Bus Selector2/1 -> TOS_ACC_TargetDxConfirm/1(Object_Dx)  "<Object_DX>"
  TOS_ACC_TargetMovingDirConfirm/1(TOS_ACC_TrgMovDir) -> Logical Operator4/2, [TOS_ACC_TrgMovDir_ObserVale]
  TOS_ACC_TargetDxConfirm/1(TOS_ACCTargetInEgoFront) -> Logical Operator4/3, [TOS_ACC_TargetDxConfirm_ObserVale]
  Bus Selector2/2 -> TOS_ACC_TargetDxConfirm/2(TOS_TLJ_SameLaneConfirm_Flag)  "<TOS_TLJ_SameLaneConfirm_Flag>"

== system PubIfDecisionTOS_MDL/TOS_20201112/TOS_2012080320/TOS/ACC/TOS_ACCCurrentLane/ACC_Object_PreConfirm/ACC_P0_P1_Object_TargPreConfirm/ACC_P0_P1_Object_TargPreConfirm/  ==
  object_MovingState : Inport
  Object_Type : Inport  Port=2
  Compare To Constant : simulink/Logic and Bit Operations/Compare To Constant  relop===  const=OFM_OBJ_TYPE_E.CAR  OutDataTypeStr=boolean
      settings: AttributesFormatString=OFM_OBJ_TYPE_E.CAR = 2
  Compare To Constant1 : simulink/Logic and Bit Operations/Compare To Constant  relop===  const=OFM_OBJ_TYPE_E.TRUCK  OutDataTypeStr=boolean
      settings: AttributesFormatString=OFM_OBJ_TYPE_E.TRUCK = 3
  Compare To Constant2 : simulink/Logic and Bit Operations/Compare To Constant  relop===  const=OFM_OBJ_MOVINGSTATE_E.MOVING  OutDataTypeStr=boolean
      settings: AttributesFormatString=OFM_OBJ_MOVINGSTATE_E.MOVING = 2
  Compare To Constant3 : simulink/Logic and Bit Operations/Compare To Constant  relop===  const=OFM_OBJ_MOVINGSTATE_E.MOVING_SLOWLY  OutDataTypeStr=boolean
      settings: AttributesFormatString=OFM_OBJ_MOVINGSTATE_E.MOVING_SLOWLY = 5
  Compare To Constant4 : simulink/Logic and Bit Operations/Compare To Constant  relop===  const=OFM_OBJ_TYPE_E.MOTORBIKE  OutDataTypeStr=boolean
      settings: AttributesFormatString=OFM_OBJ_TYPE_E.MOTORBIKE = 4
  Compare To Constant5 : simulink/Logic and Bit Operations/Compare To Constant  relop===  const=OFM_OBJ_TYPE_E.BICYCLE  OutDataTypeStr=boolean
      settings: AttributesFormatString=OFM_OBJ_TYPE_E.BICYCLE = 5
  Compare To Constant6 : simulink/Logic and Bit Operations/Compare To Constant  relop===  const=OFM_OBJ_MOVINGSTATE_E.STOPPED  OutDataTypeStr=boolean
      settings: AttributesFormatString=OFM_OBJ_MOVINGSTATE_E.STOPPED = 4
  Compare To Constant7 : simulink/Logic and Bit Operations/Compare To Constant  relop===  const=OFM_OBJ_TYPE_E.PEDESTRIAN  OutDataTypeStr=boolean
      settings: AttributesFormatString=OFM_OBJ_TYPE_E.PEDESTRIAN = 6
  Compare To Constant8 : simulink/Logic and Bit Operations/Compare To Constant  relop===  const=OFM_OBJ_TYPE_E.UNKNOWN_TYPE  OutDataTypeStr=boolean
      settings: AttributesFormatString=OFM_OBJ_TYPE_E.UNKNOWN_TYPE = 1
  Data Type Conversion : DataTypeConversion  OutDataTypeStr=Enum: OFM_OBJ_TYPE_E
  Data Type Conversion2 : DataTypeConversion  OutDataTypeStr=Enum: OFM_OBJ_MOVINGSTATE_E
  Logical Operator : Logic  AllPortsSameDT=off  OutDataTypeStr=boolean
  Logical Operator1 : Logic  Operator=OR  Inputs=6  AllPortsSameDT=off  OutDataTypeStr=boolean
  Logical Operator2 : Logic  Operator=OR  Inputs=3  AllPortsSameDT=off  OutDataTypeStr=boolean
  TOS_ACC_P0_P1_ObjType : Outport
  wires:
  Object_Type/1 -> Data Type Conversion/1
  Data Type Conversion/1 -> Compare To Constant7/1, Compare To Constant5/1, Compare To Constant4/1, Compare To Constant1/1, Compare To Constant/1, Compare To Constant8/1
  Compare To Constant3/1 -> Logical Operator2/2
  Compare To Constant2/1 -> Logical Operator2/1
  Compare To Constant6/1 -> Logical Operator2/3
  Data Type Conversion2/1 -> Compare To Constant6/1, Compare To Constant3/1, Compare To Constant2/1
  object_MovingState/1 -> Data Type Conversion2/1
  Logical Operator/1 -> Logical Operator1/1
  Compare To Constant/1 -> Logical Operator1/2
  Compare To Constant1/1 -> Logical Operator1/3
  Compare To Constant4/1 -> Logical Operator1/4
  Compare To Constant5/1 -> Logical Operator1/5
  Logical Operator2/1 -> Logical Operator/1
  Compare To Constant8/1 -> Logical Operator/2
  Logical Operator1/1 -> TOS_ACC_P0_P1_ObjType/1
  Compare To Constant7/1 -> Logical Operator1/6

== system PubIfDecisionTOS_MDL/TOS_20201112/TOS_2012080320/TOS/ACC/TOS_ACCCurrentLane/ACC_Object_PreConfirm/ACC_P0_P1_Object_TargPreConfirm/ACC_P0_P1_Object_TargPreConfirm/Overlap ==
  LM : Inport
  Bus Selector10 : BusSelector  OutputSignals=LM_LR_Line06_dDisStart,LM_LR_Line06_dDisEnd,LM_LR_Line06_fCamValid
  Bus Selector11 : BusSelector  OutputSignals=Obj_Dx,PIL_OverlapRatio,PIL_OverlapRatio_K1,PIL_OverlapRatio_K2
  Bus Selector12 : BusSelector  OutputSignals=Obj_Dx,PIL_OverlapRatio,PIL_OverlapRatio_K1,PIL_OverlapRatio_K2
  Bus Selector7 : BusSelector  OutputSignals=LM_LR_Line04_dDisStart,LM_LR_Line04_dDisEnd,LM_LR_Line04_fCamValid
  Bus Selector8 : BusSelector  OutputSignals=Obj_Dx
  Bus Selector9 : BusSelector  OutputSignals=LM_LR_Line05_dDisStart,LM_LR_Line05_dDisEnd,LM_LR_Line05_fCamValid
  Compare To Constant{1..5,14} (6 alike) : simulink/Logic and Bit Operations/Compare To Constant  relop=>=  const=P_TOS_ACC_P0_P1_TargetInFrontEgoVehicle_OverlapThre_Val  OutDataTypeStr=boolean
      settings: AttributesFormatString=P_TOS_ACC_P0_P1_TargetInFrontEgoVehicle_OverlapThre_Val = 0.1
  Compare To Constant10 : simulink/Logic and Bit Operations/Compare To Constant  relop=<  const=P_TOS_EgoFrontDxThre_70_Val  OutDataTypeStr=boolean
      settings: AttributesFormatString=P_TOS_EgoFrontDxThre_70_Val = 70
  Compare To Constant11 : simulink/Logic and Bit Operations/Compare To Constant  relop=>=  const=P_TOS_RefPoint_dx_m  OutDataTypeStr=boolean
      settings: AttributesFormatString=P_TOS_RefPoint_dx_m = 0
  Compare To Constant12 : simulink/Logic and Bit Operations/Compare To Constant  relop=<  const=P_TOS_EgoFrontDxThre_50_Val  OutDataTypeStr=boolean
      settings: AttributesFormatString=P_TOS_EgoFrontDxThre_50_Val = 50
  Compare To Constant13 : simulink/Logic and Bit Operations/Compare To Constant  relop=>=  const=P_TOS_RefPoint_dx_m  OutDataTypeStr=boolean
      settings: AttributesFormatString=P_TOS_RefPoint_dx_m = 0
  Logical Operator10 : Logic  Inputs=5  AllPortsSameDT=off  OutDataTypeStr=boolean
  Logical Operator4 : Logic  Inputs=3  AllPortsSameDT=off  OutDataTypeStr=boolean
  Logical Operator6 : Logic  Inputs=3  AllPortsSameDT=off  OutDataTypeStr=boolean
  Logical Operator7 : Logic  Inputs=3  AllPortsSameDT=off  OutDataTypeStr=boolean
  Logical Operator8 : Logic  Operator=OR  Inputs=3  AllPortsSameDT=off  OutDataTypeStr=boolean
  Logical Operator9 : Logic  Inputs=5  AllPortsSameDT=off  OutDataTypeStr=boolean
  Relational Operator : RelationalOperator  Operator=>  OutDataTypeStr=boolean  RndMeth=Simplest
  Relational Operator1 : RelationalOperator  Operator=<=  OutDataTypeStr=boolean  RndMeth=Simplest
  Relational Operator2 : RelationalOperator  Operator=>  OutDataTypeStr=boolean  RndMeth=Simplest
  Relational Operator3 : RelationalOperator  Operator=<=  OutDataTypeStr=boolean  RndMeth=Simplest
  Relational Operator4 : RelationalOperator  Operator=>  OutDataTypeStr=boolean  RndMeth=Simplest
  Relational Operator5 : RelationalOperator  Operator=<=  OutDataTypeStr=boolean  RndMeth=Simplest
  Switch : Switch  Criteria=u2 > Threshold
  Overlap : Outport
  wires:
  Compare To Constant12/1 -> Logical Operator10/2
  Relational Operator4/1 -> Logical Operator7/1
  Bus Selector8/1 -> Relational Operator5/1, Relational Operator4/1, Relational Operator3/1, Relational Operator2/1, Relational Operator1/1, Relational Operator/1  "<Obj_Dx>"
  Logical Operator4/1 -> Logical Operator8/1
  Compare To Constant11/1 -> Logical Operator9/1
  Relational Operator/1 -> Logical Operator4/1
  Bus Selector12/1 -> Compare To Constant13/1, Compare To Constant12/1  "<Obj_Dx>"
  Bus Selector9/3 -> Logical Operator6/3  "<LM_LR_Line05_fCamValid>"
  Logical Operator8/1 -> Switch/2
  Logical Operator9/1 -> Switch/1
  Relational Operator5/1 -> Logical Operator7/2
  Bus Selector7/1 -> Relational Operator/2  "<LM_LR_Line04_dDisStart>"
  Bus Selector12/3 -> Compare To Constant1/1  "<PIL_OverlapRatio_K1>"
  Bus Selector11/3 -> Compare To Constant4/1  "<PIL_OverlapRatio_K1>"
  Compare To Constant5/1 -> Logical Operator9/5
  Logical Operator6/1 -> Logical Operator8/2
  Relational Operator2/1 -> Logical Operator6/1
  Compare To Constant13/1 -> Logical Operator10/1
  Relational Operator3/1 -> Logical Operator6/2
  Bus Selector11/4 -> Compare To Constant5/1  "<PIL_OverlapRatio_K2>"
  Bus Selector11/1 -> Compare To Constant10/1, Compare To Constant11/1  "<Obj_Dx>"
  Compare To Constant10/1 -> Logical Operator9/2
  Bus Selector9/2 -> Relational Operator3/2  "<LM_LR_Line05_dDisEnd>"
  Bus Selector9/1 -> Relational Operator2/2  "<LM_LR_Line05_dDisStart>"
  Bus Selector10/1 -> Relational Operator4/2  "<LM_LR_Line06_dDisStart>"
  Compare To Constant4/1 -> Logical Operator9/4
  Bus Selector7/2 -> Relational Operator1/2  "<LM_LR_Line04_dDisEnd>"
  Bus Selector10/2 -> Relational Operator5/2  "<LM_LR_Line06_dDisEnd>"
  LM/1 -> Bus Selector12/1, Bus Selector10/1, Bus Selector9/1, Bus Selector7/1, Bus Selector8/1, Bus Selector11/1
  Bus Selector10/3 -> Logical Operator7/3  "<LM_LR_Line06_fCamValid>"
  Bus Selector7/3 -> Logical Operator4/3  "<LM_LR_Line04_fCamValid>"
  Relational Operator1/1 -> Logical Operator4/2
  Switch/1 -> Overlap/1
  Compare To Constant3/1 -> Logical Operator9/3
  Compare To Constant14/1 -> Logical Operator10/3
  Bus Selector11/2 -> Compare To Constant3/1  "<PIL_OverlapRatio>"
  Logical Operator7/1 -> Logical Operator8/3
  Bus Selector12/4 -> Compare To Constant2/1  "<PIL_OverlapRatio_K2>"
  Compare To Constant2/1 -> Logical Operator10/5
  Bus Selector12/2 -> Compare To Constant14/1  "<PIL_OverlapRatio>"
  Compare To Constant1/1 -> Logical Operator10/4
  Logical Operator10/1 -> Switch/3

== system PubIfDecisionTOS_MDL/TOS_20201112/TOS_2012080320/TOS/ACC/TOS_ACCCurrentLane/ACC_Object_PreConfirm/ACC_P0_P1_Object_TargPreConfirm/ACC_P0_P1_Object_TargPreConfirm/Subsystem ==
  PP_ObjFusType_FC_FR_Confirm : Inport
  PP_ObjFusType_FR_Confirm : Inport  Port=2
  PP_ObjFusType_FC_Confirm : Inport  Port=3
  Compare To Constant1 : simulink/Logic and Bit Operations/Compare To Constant  relop===  const=C_TOS_PP_ObjFusType_FC_Confirm_b  OutDataTypeStr=boolean
      settings: AttributesFormatString=C_TOS_PP_ObjFusType_FC_Confirm_b = 1
  Compare To Constant5 : simulink/Logic and Bit Operations/Compare To Constant  relop===  const=C_TOS_PP_ObjFusType_FC_FR_Confirm_b  OutDataTypeStr=boolean
      settings: AttributesFormatString=C_TOS_PP_ObjFusType_FC_FR_Confirm_b = 1
  Compare To Constant6 : simulink/Logic and Bit Operations/Compare To Constant  relop===  const=C_TOS_PP_ObjFusType_FR_Confirm_b  OutDataTypeStr=boolean
      settings: AttributesFormatString=C_TOS_PP_ObjFusType_FR_Confirm_b = 1
  Logical Operator : Logic  Operator=OR  Inputs=3  AllPortsSameDT=off  OutDataTypeStr=boolean
  TOS_ACC_P0_P1_TargetPre_TargetFusionTypeFlag : Outport
  wires:
  Logical Operator/1 -> TOS_ACC_P0_P1_TargetPre_TargetFusionTypeFlag/1
  Compare To Constant1/1 -> Logical Operator/3
  Compare To Constant6/1 -> Logical Operator/2
  PP_ObjFusType_FC_FR_Confirm/1 -> Compare To Constant5/1
  PP_ObjFusType_FC_Confirm/1 -> Compare To Constant1/1
  PP_ObjFusType_FR_Confirm/1 -> Compare To Constant6/1
  Compare To Constant5/1 -> Logical Operator/1

== system PubIfDecisionTOS_MDL/TOS_20201112/TOS_2012080320/TOS/ACC/TOS_ACCCurrentLane/ACC_Object_PreConfirm/ACC_P0_P1_Object_TargPreConfirm/ACC_P0_P1_Object_TargPreConfirm/Subsystem1 ==
  note: 目标分裂处理
  FR_Confirm : Inport
  Obj_MovingState : Inport  Port=2
  Obj_Dx : Inport  Port=3
  ACC_TargetP0_ID_K1 : Inport  Port=4
  ACC_TargetP0_Dx_K1 : Inport  Port=5
  Object_ID : Inport  Port=6
  Add : Sum
  Compare To Constant : simulink/Logic and Bit Operations/Compare To Constant  relop=~=  const=C_TOS_OFMObjIDInvilad_Val  OutDataTypeStr=boolean
      settings: AttributesFormatString=C_TOS_OFMObjIDInvilad_Val = 0
  Compare To Constant1 : simulink/Logic and Bit Operations/Compare To Constant  relop===  const=C_TOS_PP_ObjFusType_FR_Confirm_b  OutDataTypeStr=boolean
      settings: AttributesFormatString=C_TOS_PP_ObjFusType_FR_Confirm_b = 1
  Compare To Constant2 : simulink/Logic and Bit Operations/Compare To Constant  relop===  const=OFM_OBJ_MOVINGSTATE_E.UNKNOWN  OutDataTypeStr=boolean
      settings: AttributesFormatString=OFM_OBJ_MOVINGSTATE_E.UNKNOWN = 1
  Compare To Constant3 : simulink/Logic and Bit Operations/Compare To Constant  relop===  const=OFM_OBJ_MOVINGSTATE_E.INVALID  OutDataTypeStr=boolean
      settings: AttributesFormatString=OFM_OBJ_MOVINGSTATE_E.INVALID = 0
  Compare To Constant4 : simulink/Logic and Bit Operations/Compare To Constant  relop===  const=OFM_OBJ_MOVINGSTATE_E.STATIONARY  OutDataTypeStr=boolean
      settings: AttributesFormatString=OFM_OBJ_MOVINGSTATE_E.STATIONARY = 3
  Constant : Constant  OutDataTypeStr=single
  Constant1 : Constant  Value=0  OutDataTypeStr=boolean
  Constant2 : Constant  Value=0  OutDataTypeStr=boolean
  Data Type Conversion1 : DataTypeConversion  OutDataTypeStr=Enum: OFM_OBJ_MOVINGSTATE_E
  Logical Operator : Logic  Operator=OR  Inputs=3  AllPortsSameDT=off  OutDataTypeStr=boolean
  Logical Operator1 : Logic  AllPortsSameDT=off  OutDataTypeStr=boolean
  Logical Operator2 : Logic  AllPortsSameDT=off  OutDataTypeStr=boolean
  Relational Operator : RelationalOperator  Operator=<  OutDataTypeStr=boolean  RndMeth=Simplest
  Relational Operator1 : RelationalOperator  Operator=~=  OutDataTypeStr=boolean  RndMeth=Simplest
  Switch : Switch  Criteria=u2 ~= 0
  Switch1 : Switch  Criteria=u2 ~= 0
  TOS_ACC_P0_P1_TargetPre_ObjectPassedbyTarget_Flag : Outport
  wires:
  Switch/1 -> TOS_ACC_P0_P1_TargetPre_ObjectPassedbyTarget_Flag/1
  Compare To Constant3/1 -> Logical Operator/1
  Compare To Constant/1 -> Logical Operator2/1
  Constant/1 -> Add/2
  Obj_MovingState/1 -> Data Type Conversion1/1
  Obj_Dx/1 -> Relational Operator/1
  Relational Operator/1 -> Switch1/1
  Compare To Constant1/1 -> Logical Operator1/1
  Compare To Constant2/1 -> Logical Operator/2
  FR_Confirm/1 -> Compare To Constant1/1
  Logical Operator1/1 -> Switch1/2
  Switch1/1 -> Switch/1
  Add/1 -> Relational Operator/2
  Logical Operator/1 -> Logical Operator1/2
  Constant2/1 -> Switch/3
  ACC_TargetP0_Dx_K1/1 -> Add/1
  Constant1/1 -> Switch1/3
  Compare To Constant4/1 -> Logical Operator/3
  ACC_TargetP0_ID_K1/1 -> Relational Operator1/1, Compare To Constant/1
  Data Type Conversion1/1 -> Compare To Constant4/1, Compare To Constant2/1, Compare To Constant3/1
  Object_ID/1 -> Relational Operator1/2
  Relational Operator1/1 -> Logical Operator2/2
  Logical Operator2/1 -> Switch/2

== system PubIfDecisionTOS_MDL/TOS_20201112/TOS_2012080320/TOS/ACC/TOS_ACCCurrentLane/ACC_Object_PreConfirm/ACC_P0_P1_Object_TargPreConfirm/ACC_P0_P1_Object_TargPreConfirm/Subsystem2 ==
  <PP_REElementType> : Inport
  Compare To Constant1 : simulink/Logic and Bit Operations/Compare To Constant  relop===  const=C_TOS_ObjNotREElementType  OutDataTypeStr=boolean
      settings: AttributesFormatString=%<const> = 0
  TOS_ACC_P0_P1_REElementType : Outport
  wires:
  Compare To Constant1/1 -> TOS_ACC_P0_P1_REElementType/1
  <PP_REElementType>/1 -> Compare To Constant1/1

== system PubIfDecisionTOS_MDL/TOS_20201112/TOS_2012080320/TOS/ACC/TOS_ACCCurrentLane/ACC_Object_PreConfirm/ACC_P0_P1_Object_TargPreConfirm/ACC_P0_P1_Object_TargPreConfirm/Subsystem3 ==
  FR_Confirm : Inport
  Obj_MovingState : Inport  Port=2
  Object_ObstacleProb : Inport  Port=3
  Object_DY : Inport  Port=4
  Chart : Stateflow chart  TreatAsAtomicUnit=on
  Data Type Conversion1 : DataTypeConversion  OutDataTypeStr=Enum: OFM_OBJ_MOVINGSTATE_E
  TOS_ACC_P0_P1_TargetPre_FenceFlag : Outport
  wires:
  Chart/1(ObjectisFence_Flag) -> TOS_ACC_P0_P1_TargetPre_FenceFlag/1
  Object_DY/1 -> Chart/4(Object_DY)
  FR_Confirm/1 -> Chart/1(FR_Confirm)
  Obj_MovingState/1 -> Data Type Conversion1/1
  Object_ObstacleProb/1 -> Chart/3(Object_ObstacleProb)
  Data Type Conversion1/1 -> Chart/2(Obj_MovingState)
